simulink model "TTypeInverter_R2022a"  (R2022a)
settings: Solver=ode23t  StartTime=0.0  StopTime=0.2  RelTol=1e-3  EnableMultiTasking=on
values from neighbouring files (symbols this model uses):
  C_c = 30*10^-6    (= 3e-05)    [TTypeInverterVals.m]
  den = abs(G_pr_r_z.Denominator{1,1})    [TTypeInverterVals.m]
  den15 = abs(G_pr_r_15_z.Denominator{1,1})    [TTypeInverterVals.m]
  den21 = abs(G_pr_r_21_z.Denominator{1,1})    [TTypeInverterVals.m]
  den5 = abs(G_pr_r_5_z.Denominator{1,1})    [TTypeInverterVals.m]
  den7 = abs(G_pr_r_7_z.Denominator{1,1})    [TTypeInverterVals.m]
  f_o = 50    [TTypeInverterVals.m]
  G_diff_z = c2d(G_diff_s,Ts,opt)    [ControllerDesign.m]    (also in TTypeInverterVals.m = c2d(G_diff_s,Ts,'foh'))
  Kc = 2.5    [ControllerDesign.m]    (also in TTypeInverterVals.m)
  Klim = 5    [TTypeInverterVals.m]
  Kp = 1/mag/(10^(1.14/20))    [ControllerDesign.m]    (also in TTypeInverterVals.m = 0.9444)
  Kr = omega_c_o/2    (= 3141.59265359)    [ControllerDesign.m]    (also in TTypeInverterVals.m)
  N = 26    [Inductance.m]    (also in TTypeInverterVals.m = [0])
  num = abs(G_pr_r_z.Numerator{1,1})    [TTypeInverterVals.m]
  num15 = abs(G_pr_r_15_z.Numerator{1,1})    [TTypeInverterVals.m]
  num21 = abs(G_pr_r_21_z.Numerator{1,1})    [TTypeInverterVals.m]
  num5 = abs(G_pr_r_5_z.Numerator{1,1})    [TTypeInverterVals.m]
  num7 = abs(G_pr_r_7_z.Numerator{1,1})    [TTypeInverterVals.m]
  omega_o = fo*2*pi    (= 314.159265359)    [ControllerDesign.m]    (also in TTypeInverterVals.m)
  omega_w = 0.1*2*pi    (= 0.628318530718)    [ControllerDesign.m]    (also in TTypeInverterVals.m)
  pr_sat_val = ceil(3*io_nom)    [TTypeInverterVals.m]
  Q = eye(3)    [TTypeInverterVals.m]
  R = [R_iL 0 ... (first row only)    [TTypeInverterVals.m]
  R_l_20p = Vout^2/P_lin_20p    (= 10.58)    [TTypeInverterVals.m]
  R_l_3p = Vout/(P_max_3p/(Vout*3))    (= 2.116)    [TTypeInverterVals.m]
  R_l_80p = Vout^2/P_lin_80p    (= 2.645)    [TTypeInverterVals.m]
  R_l_nl = Vout^2/P_lin    (= 3.11176470588)    [TTypeInverterVals.m]
  R_l_nl_3p = Vout_3p^2/P_lin_3p    [TTypeInverterVals.m]
  R_Lc = 5.6e-3    (= 0.0056)    [TTypeInverterVals.m]
  R_nl_load = Uc^2/(0.66*S_tot)    (= 14.9121893939)    [TTypeInverterVals.m]
  R_nl_load_3p = Uc_3p^2/(0.66*S_tot_3p)    (= 4.97072979798)    [TTypeInverterVals.m]
  R_nl_s = 0.04*Vout^2/S_tot    (= 0.2645)    [TTypeInverterVals.m]
  R_nl_s_3p = 0.04*Vout_3p^2/S_tot_3p    [TTypeInverterVals.m]
  T_sw = 1/f_sw    (= 4.16666666667e-05)    [TTypeInverterVals.m]
  Tcomp = Ts/4    (= 2.60400009204e-06)    [TTypeInverterVals.m]
  Ts = 1/fs    (= 1.04166666667e-05)    [ControllerDesign.m]    (also in KalmanFilter.m = 2.08333333333e-05; TTypeInverterVals.m = 1.04160003681e-05)
  VDC = 800    [TTypeInverterVals.m]
  Vout_amp = Vout*sqrt(2)    [TTypeInverterVals.m]
undefined symbols (not defined in the file or in its folder): a0, a1, b0, b1, Discrete, G_ll_z, Ki, Kpc, KT, kv, Time, UKF_data
libraries: ee_lib x94, nesl_utility x48, fl_lib x39, dspstat3 x15, spsTriangleGeneratorLib x6, ctrlSharedLib x3, spsRMSLib x3, spsTHDLib x3
(part 1 of 5)
settings Model: Creator=sebastian  LastModifiedBy=sebastian
settings DataIOCC: ReturnWorkspaceOutputs=off
settings SimscapeCC: SimscapeNormalizeSystem=off

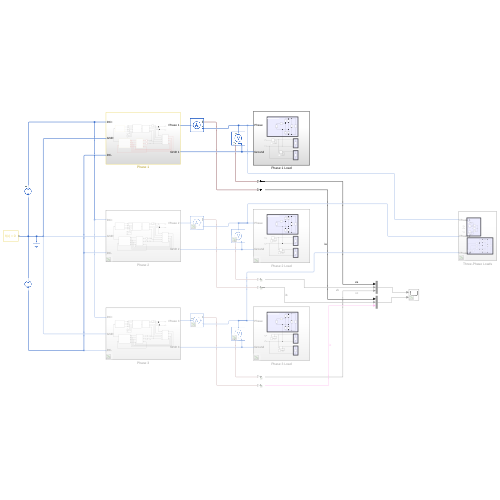
[thumbnail: Simulink's stored preview of the top-level diagram]
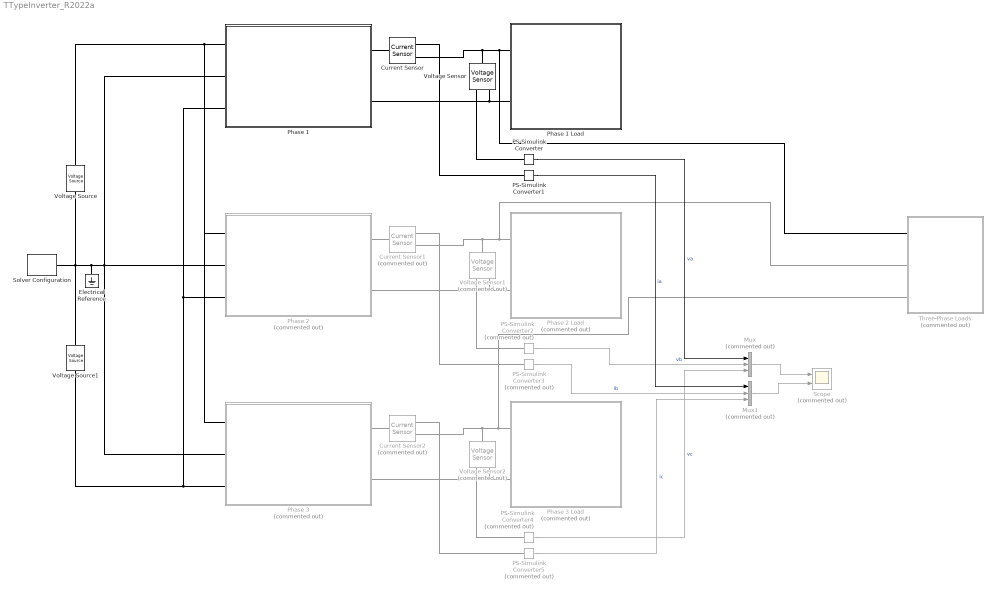
== system TTypeInverter_R2022a ==
  Current Sensor : fl_lib/Electrical/Electrical Sensors/Current Sensor
      settings: SourceProductBaseCode=PW,SS,VE
  Current Sensor1 : fl_lib/Electrical/Electrical Sensors/Current Sensor  Commented=on
      settings: SourceProductBaseCode=PW,SS,VE
  Current Sensor2 : fl_lib/Electrical/Electrical Sensors/Current Sensor  Commented=on
      settings: SourceProductBaseCode=PW,SS,VE
  Electrical Reference : fl_lib/Electrical/Electrical Elements/Electrical Reference
      settings: SourceProductBaseCode=PW,SS,VE
  Mux : Mux  Commented=on  Inputs=3
  Mux1 : Mux  Commented=on  Inputs=3
  PS-Simulink Converter : nesl_utility/PS-Simulink Converter  PhysicalDomain=network_engine_domain  SubClassName=ps_output  LeftPortType=input  RightPortType=output  PseudoPeriodic=off  Frequencies=[]  VectorFormat=inherit  Unit=inherit  AffineConversion=off
      settings: SourceProductBaseCode=SS,PW,VE
  PS-Simulink Converter1 : nesl_utility/PS-Simulink Converter  PhysicalDomain=network_engine_domain  SubClassName=ps_output  LeftPortType=input  RightPortType=output  PseudoPeriodic=off  Frequencies=[]  VectorFormat=inherit  Unit=inherit  AffineConversion=off
      settings: SourceProductBaseCode=SS,PW,VE
  PS-Simulink Converter{2..5} (4 alike) : nesl_utility/PS-Simulink Converter  Commented=on  PhysicalDomain=network_engine_domain  SubClassName=ps_output  LeftPortType=input  RightPortType=output  PseudoPeriodic=off  Frequencies=[]  VectorFormat=inherit  Unit=inherit  AffineConversion=off
      settings: SourceProductBaseCode=SS,PW,VE
  Phase 1 : Subsystem
  Phase 1 Load : Subsystem
  Phase 2 : Subsystem  Commented=on
  Phase 2 Load : Subsystem  Commented=on
  Phase 3 : Subsystem  Commented=on
  Phase 3 Load : Subsystem  Commented=on
  Scope : Scope  Commented=on  NumInputPorts=2
  Solver Configuration : nesl_utility/Solver Configuration  PhysicalDomain=network_engine_domain  SubClassName=solver  LeftPortType=input  RightPortType=generic  Tones=[]  Harmonics=[]  SimulateNoise=off  Profile=off  UseLocalSampling=off  EnableSwitchedLinearOptims=on  FrequencyDomain=off  UseCCode=off  RelTol=0.001  AbsTol=0.001  MinStep=1e-09  ToWorkspace=off  RevertToSquareIcSolve=off  NumHomotopyIterations=100  PhasorMode=off  PhasorModeNumHarmonics=1  IndexReductionMethod=DerivativeReplacement  DoDC=off  ResidualTolerance=1e-09  UseLocalSolver=off  LocalSolverChoice=NE_BACKWARD_EULER_ADVANCER  LocalSolverSampleTime=Ts/10000  DoFixedCost=off  MaxNonlinIter=3  MaxModeIter=2  ComputeImpulses=off  ImpulseIterations=2  LinearAlgebra=auto  LinearAlgebraNumThread=0  EquationFormulation=NE_TIME_EF  DelaysMemoryBudget=1024  AutomaticFiltering=on  FilteringTimeConstant=0.001  PartitionStorageMethod=AS_NEEDED  PartitionMemoryBudget=1024  PartitionMethod=ROBUST
      settings: SourceProductBaseCode=SS,PW,VE
  Three-Phase Loads : Subsystem  Commented=on
  Voltage Sensor : fl_lib/Electrical/Electrical Sensors/Voltage Sensor
      settings: SourceProductBaseCode=PW,SS,VE
  Voltage Sensor1 : fl_lib/Electrical/Electrical Sensors/Voltage Sensor  Commented=on
      settings: SourceProductBaseCode=PW,SS,VE
  Voltage Sensor2 : fl_lib/Electrical/Electrical Sensors/Voltage Sensor  Commented=on
      settings: SourceProductBaseCode=PW,SS,VE
  Voltage Source : ee_lib/Sources/Voltage Source  dc_voltage=VDC/2 V  ac_voltage=0 V  ac_shift=0 rad  ac_frequency=60 Hz  noise_mode=1  PSD=0.0001 V^2/Hz  repeatability=3  auto_seed=3437178441  user_seed=0  sample_time=Ts s  i_specify=off  i_priority=None  i=0 A  i_nominal_specify=off  i_nominal_unit=A  i_nominal_value=1  v_specify=off  v_priority=None  v=0 V  v_nominal_specify=off  v_nominal_unit=V  v_nominal_value=1
  Voltage Source1 : ee_lib/Sources/Voltage Source  dc_voltage=VDC/2 V  ac_voltage=0 V  ac_shift=0 rad  ac_frequency=60 Hz  noise_mode=1  PSD=0.0001 V^2/Hz  repeatability=3  auto_seed=609397185  user_seed=0  sample_time=Ts s  i_specify=off  i_priority=None  i=0 A  i_nominal_specify=off  i_nominal_unit=A  i_nominal_value=1  v_specify=off  v_priority=None  v=0 V  v_nominal_specify=off  v_nominal_unit=V  v_nominal_value=1
  wires:
  Mux/1 -> Scope/1
  Mux1/1 -> Scope/2
  PS-Simulink Converter/1 -> Mux/1  "va"
  PS-Simulink Converter2/1 -> Mux/2  "vb"
  PS-Simulink Converter4/1 -> Mux/3  "vc"
  PS-Simulink Converter1/1 -> Mux1/1  "ia"
  PS-Simulink Converter3/1 -> Mux1/2  "ib"
  PS-Simulink Converter5/1 -> Mux1/3  "ic"
  connections:
  Phase 1 Load/LConn2 -- Voltage Sensor/RConn2 -- Phase 1/RConn2
  Solver Configuration/RConn1 -- Phase 2/LConn2 -- Phase 3/LConn2 -- Phase 1/LConn2 -- Electrical Reference/LConn1 -- Voltage Source/RConn1 -- Voltage Source1/LConn1
  Voltage Source/LConn1 -- Phase 3/LConn1 -- Phase 2/LConn1 -- Phase 1/LConn1
  Phase 1/LConn3 -- Voltage Source1/RConn1 -- Phase 3/LConn3 -- Phase 2/LConn3
  Current Sensor/LConn1 -- Phase 1/RConn1
  Current Sensor/RConn2 -- Voltage Sensor/LConn1 -- Three-Phase Loads/LConn1 -- Phase 1 Load/LConn1
  PS-Simulink Converter/LConn1 -- Voltage Sensor/RConn1
  Current Sensor/RConn1 -- PS-Simulink Converter1/LConn1
  Current Sensor1/RConn2 -- Voltage Sensor1/LConn1 -- Three-Phase Loads/LConn2 -- Phase 2 Load/LConn1
  Phase 2 Load/LConn2 -- Voltage Sensor1/RConn2 -- Phase 2/RConn2
  PS-Simulink Converter2/LConn1 -- Voltage Sensor1/RConn1
  Current Sensor1/LConn1 -- Phase 2/RConn1
  Current Sensor1/RConn1 -- PS-Simulink Converter3/LConn1
  Current Sensor2/RConn2 -- Voltage Sensor2/LConn1 -- Three-Phase Loads/LConn3 -- Phase 3 Load/LConn1
  Phase 3 Load/LConn2 -- Voltage Sensor2/RConn2 -- Phase 3/RConn2
  PS-Simulink Converter4/LConn1 -- Voltage Sensor2/RConn1
  Current Sensor2/LConn1 -- Phase 3/RConn1
  Current Sensor2/RConn1 -- PS-Simulink Converter5/LConn1

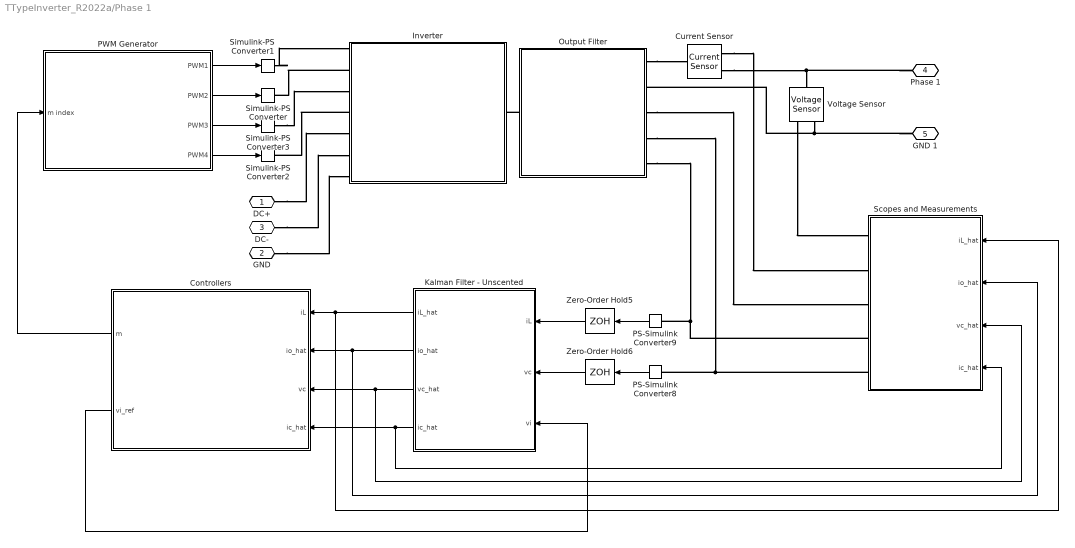
== system TTypeInverter_R2022a/Phase 1 ==
  Controllers : Subsystem
  Current Sensor : fl_lib/Electrical/Electrical Sensors/Current Sensor
      settings: SourceProductBaseCode=PW,SS,VE
  Inverter : Subsystem
  Kalman Filter - Unscented : Subsystem
  Output Filter : Subsystem
  PS-Simulink Converter8 : nesl_utility/PS-Simulink Converter  PhysicalDomain=network_engine_domain  SubClassName=ps_output  LeftPortType=input  RightPortType=output  PseudoPeriodic=off  Frequencies=[]  VectorFormat=inherit  Unit=inherit  AffineConversion=off
      settings: SourceProductBaseCode=SS,PW,VE
  PS-Simulink Converter9 : nesl_utility/PS-Simulink Converter  PhysicalDomain=network_engine_domain  SubClassName=ps_output  LeftPortType=input  RightPortType=output  PseudoPeriodic=off  Frequencies=[]  VectorFormat=inherit  Unit=inherit  AffineConversion=off
      settings: SourceProductBaseCode=SS,PW,VE
  PWM Generator : Subsystem
  Scopes and Measurements : Subsystem
      settings: PortSchema="{\"entries\":[{\"content\":{\"sides\":[{\"content\":{\"connectorIds\":[\"LConn1\",\"LConn2\",\"LConn3\",\"LConn4\",\"LConn5\"]},\"type\":\"ConnectorPlacement.EquallySpacedRectSide\",\"uuid\":\"9cb3f6d1-a698-4256-82c6-cde7349a629b\"},{\"content\":{\"connectorIds\":[\"In1\",\"In2\",\"In3\",\"In4\"],\"side\":\"RIGHT\"},\"type\":\"ConnectorPlacement.EquallySpacedRectSide\",\"uuid\":\"1e882b0f-d5eb-4cef-9b33-a811b5aef736\"},{\"content\":{\"connectorIds\":[],\"side\":\"TOP\"},\"type\":\"ConnectorPlacement.EquallySpacedRectSide\",\"uuid\":\"e9e8da66-95e1-4884-9361-97f2ef91d9a4\"}]},\"type\":\"ConnectorPlacement.EquallySpacedConnector\",\"uuid\":\"50359238-0e1d-4354-ac1b-c407791d07c2\"}],\"packageUris\":[\"http://schema.mathworks.com/mf0/Connector/R2020b\"],\"version\":\"1.0\"}"
  Simulink-PS Converter{,1..3} (4 alike) : nesl_utility/Simulink-PS Converter  PhysicalDomain=network_engine_domain  SubClassName=ps_input  LeftPortType=input  RightPortType=output  PseudoPeriodic=off  Frequencies=[]  NoiseDistribution=none  NoiseParameters=[]  Unit=1  AffineConversion=off  FilteringAndDerivatives=provide  SimscapeFilterOrder=1  InputFilterTimeConstant=0.001  UdotUserProvided=0
      settings: SourceProductBaseCode=SS,PW,VE
  Voltage Sensor : fl_lib/Electrical/Electrical Sensors/Voltage Sensor
      settings: SourceProductBaseCode=PW,SS,VE
  Zero-Order Hold5 : ZeroOrderHold  SampleTime=Ts
  Zero-Order Hold6 : ZeroOrderHold  SampleTime=Ts
  DC+ : PMIOPort  Side=Left
  GND : PMIOPort  Port=2  Side=Left
  DC- : PMIOPort  Port=3  Side=Left
  Phase 1 : PMIOPort  Port=4  Side=Right
  GND 1 : PMIOPort  Port=5  Side=Right
  wires:
  PS-Simulink Converter8/1 -> Zero-Order Hold6/1
  Kalman Filter - Unscented/1(iL_hat) -> Controllers/1(iL), Scopes and Measurements/1(iL_hat)
  PWM Generator/4(PWM4) -> Simulink-PS Converter2/1
  Controllers/2(vi_ref) -> Kalman Filter - Unscented/3(vi)
  Kalman Filter - Unscented/3(vc_hat) -> Scopes and Measurements/3(vc_hat), Controllers/3(vc)
  Zero-Order Hold5/1 -> Kalman Filter - Unscented/1(iL)
  PS-Simulink Converter9/1 -> Zero-Order Hold5/1
  Controllers/1(m) -> PWM Generator/1(m index)
  PWM Generator/2(PWM2) -> Simulink-PS Converter/1
  Zero-Order Hold6/1 -> Kalman Filter - Unscented/2(vc)
  PWM Generator/1(PWM1) -> Simulink-PS Converter1/1
  PWM Generator/3(PWM3) -> Simulink-PS Converter3/1
  Kalman Filter - Unscented/2(io_hat) -> Scopes and Measurements/2(io_hat), Controllers/2(io_hat)
  Kalman Filter - Unscented/4(ic_hat) -> Scopes and Measurements/4(ic_hat), Controllers/4(ic_hat)
  connections:
  Simulink-PS Converter3/RConn1 -- Inverter/LConn3
  Simulink-PS Converter1/RConn1 -- Inverter/LConn1
  Output Filter/RConn3 -- Scopes and Measurements/LConn3
  Voltage Sensor/RConn2 -- GND 1/RConn1 -- Output Filter/RConn2
  Voltage Sensor/RConn1 -- Scopes and Measurements/LConn1
  Current Sensor/RConn2 -- Phase 1/RConn1 -- Voltage Sensor/LConn1
  Inverter/LConn4 -- Simulink-PS Converter2/RConn1
  Output Filter/RConn5 -- Scopes and Measurements/LConn4 -- PS-Simulink Converter9/LConn1
  Output Filter/LConn1 -- Inverter/RConn1
  Current Sensor/RConn1 -- Scopes and Measurements/LConn2
  Inverter/LConn2 -- Simulink-PS Converter/RConn1
  Output Filter/RConn4 -- Scopes and Measurements/LConn5 -- PS-Simulink Converter8/LConn1
  Output Filter/RConn1 -- Current Sensor/LConn1
  DC+/RConn1 -- Inverter/LConn5
  DC-/RConn1 -- Inverter/LConn6
  GND/RConn1 -- Inverter/LConn7

== system TTypeInverter_R2022a/Phase 1 Load ==
  note: Capacitor may be pre-charged to 290V!
  note: Reference test load
  note: Reference nonlinear load
  note: 20% Load
  note: 80% Load
  Capacitor4 : ee_lib/Passive/Capacitor  cap_option=0  c=C_nl F  Cvec=[1e-05, 1e-06] F  Vvec=[0, 10] V  CV_table_symmetry=1  f_vec=[1, 10] kHz  DFext_vec=[.8, 1.2]  enable_C_tol=0  C_tol=5  tol_distribution=1  nSigma=4  r=R_C_nl Ohm  g=0 1/Ohm  averaging_period=0 s  enable_operating_limits=0  operating_limit_action=2  max_working_voltage_range=[-25, 25] V  power_rating=1 W  enable_faults=0  fault_action=1  Cscale_faulted=100  R_faulted=1e-3 Ohm  G_faulted=0 1/Ohm  tau_fault=1e-3 s  enable_temporal_fault=0  t_fault=1 s  enable_behavioral_fault=0  max_permissible_voltage_range=[-100, 100] V  t_fail_on_voltage=1 s  i_specify=off  i_priority=None  i=0 A  i_nominal_specify=off  i_nominal_unit=A  i_nominal_value=1  v_specify=off  v_priority=High  v=325 V  v_nominal_specify=off  v_nominal_unit=V  v_nominal_value=325  vc_specify=off  vc_priority=High  vc=290 V  vc_nominal_specify=off  vc_nominal_unit=V  vc_nominal_value=325
  Diode{1..4} (4 alike) : ee_lib/Semiconductors & Converters/Diode  ModelType=ee.enum.diode.modelType.pwl  TableType=ee.enum.diode.tableType.IfMat  IfMat=[.07, .12, .19, 1.75, 4.24, 7.32, 11.2; .16, .3, .72, 2.14, 5.02, 8.35, 13.12] A  VfMat=[.9, 1.15, 1.25, 1.5, 1.75, 2.17, 2.6, 2.85; .58, .68, .75, 1.1, 1.38, 1.77, 2.27, 2.7] V  TjVec=[25, 125] degC  VfVec=[.5, .7, .9, 1.3, 1.7, 2.1, 2.5] V  IfVec=[.1, .2, .5, 1, 2, 4, 7, 10] A  Vf=V_f V  Ron=R_d Ohm  Goff=1e-8 S  prmExp=ee.enum.diode.expParam.useTwo  I12=[.0137, .545] A  V12=[.6, .7] V  RS=0 Ohm  Tmeas=25 degC  IS=1e-12 A  ec=1  I1=0.0137 A  V1=0.6 V  N_series=1  N_parallel=1  Rz=0.3 Ohm  BV=inf V  C_param=ee.enum.diode.capParam.fixed  CJ=5 pF  CJ0=5 pF  Vvec=[.1, 10, 100] V  Cvec=[3.5, 1, .4] pF  VJ=1 V  Mgrad=0.5  FC=0.5  Q_param=ee.enum.diode.recoveryParam.off  iRM=-7.15 A  iF=4 A  didt=-750 A/us  trr_factor=3  trr=115 ns  Qrr=150 nA*s  Vr=-600 V  Ls=150 nH  Erec=0.03 J  TT=50 ns  tau=100 ns  T_param=ee.enum.diode.temperatureParam.off  Tdevice=25 degC  I1_T2=0.245 A  V1_T2=0.5 V  IS_T2=1.25e-7 A  Tmeas2=125 degC  XTI_param=ee.enum.diode.xtiParam.pn  XTI=3  EG_param=ee.enum.diode.egapParam.material_si  EG=1.11 eV  dBVdT=0 V/K  enable_faults=simscape.enum.onoff.off  fault_action=simscape.enum.assert.action.none  fault_types=ee.enum.diode.faults.open  tau_fault=1e-3 s  IfMat_faulted=[.07, .12, .19, 1.75, 4.24, 7.32, 11.2; .16, .3, .72, 2.14, 4.02, 6.35, 9.12] A  VfMat_faulted=[.9, 1.15, 1.25, 1.5, 1.75, 2.17, 2.6, 2.85; .58, .68, .75, 1.1, 1.38, 1.77, 2.27, 2.7] V  VfVec_faulted=[.5, .7, .9, 1.3, 1.7, 2.1, 2.5] V  IfVec_faulted=[.1, .2, .5, 1, 2, 4, 7, 10] A  Ropen_faulted=1000 Ohm  Gshort_faulted=1000 1/Ohm  Vf_faulted=0.6 V  Ron_faulted=0.3 Ohm  Goff_faulted=1e-8 S  I12_faulted=[.0137, .545] A  V12_faulted=[.6, .7] V  IS_faulted=1e-12 A  ec_faulted=1  I1_faulted=0.0137 A  V1_faulted=0.6 V  RS_faulted=0 Ohm  Rz_faulted=0.3 Ohm  BV_faulted=inf V  Cscale_faulted=100  enable_temporal_fault=simscape.enum.onoff.off  t_fault=inf s  enable_behavioral_fault=simscape.enum.onoff.off  max_permissible_voltage=inf V  n_fail_on_voltage=1  max_permissible_current=inf A  t_fail_on_current=1 s  max_permissible_dVdt=inf V/s  enable_fault_input=simscape.enum.onoff.off  i_specify=off  i_priority=None  i=0 A  i_nominal_specify=off  i_nominal_unit=A  i_nominal_value=1  v_specify=off  v_priority=None  v=0 V  v_nominal_specify=off  v_nominal_unit=V  v_nominal_value=1  i_diode_specify=off  i_diode_priority=None  i_diode=0 A  i_diode_nominal_specify=off  i_diode_nominal_unit=A  i_diode_nominal_value=1  v_diode_specify=off  v_diode_priority=None  v_diode=0 V  v_diode_nominal_specify=off  v_diode_nominal_unit=V  v_diode_nominal_value=1  i_capacitor_specify=off  i_capacitor_priority=None  i_capacitor=0 A  i_capacitor_nominal_specify=off  i_capacitor_nominal_unit=A  i_capacitor_nominal_value=1  v_capacitor_specify=off  v_capacitor_priority=None  v_capacitor=0 V  v_capacitor_nominal_specify=off  v_capacitor_nominal_unit=V  v_capacitor_nominal_value=1  power_dissipated_specify=off  power_dissipated_priority=None  power_dissipated=0 W  power_dissipated_nominal_specify=off  power_dissipated_nominal_unit=W  power_dissipated_nominal_value=1  max_permissible_temperature=inf K  t_fail_on_temperature=1 s  thermal_network_parameterization=ee.enum.thermalNetworkTopology.junctionCase  Rth=[0, 10] K/W  Rth_Cauer=[1, 3, 10] K/W  Rth_Foster=[4, 6] K/W  thermal_mass_parameterization=ee.enum.thermalNetwork.timeconstant  thermal_mass=[0, 1] J/K  thermal_mass_Cauer=[.1, .3, 1] J/K  thermal_mass_Foster=[1.5, 3] J/K  thermal_time_constant=[0, 10] s  thermal_time_constant_Cauer=[1, 3, 10] s  thermal_time_constant_Foster=[6, 18] s  thermal_mass_initial_temperatures=[25, 25] degC  thermal_mass_initial_temperatures_Cauer=[25, 25, 25] degC  steadyState_Foster=simscape.enum.onoff.on  Tvec_initial_Foster=[25, 25, 25, 25] degC
  Line Resistor : ee_lib/Passive/Resistor  R=R_nl_s Ohm  enable_R_tol=0  R_tol=5  tol_distribution=1  nSigma=4  enable_operating_limits=0  operating_limit_action=2  max_working_voltage=100 V  power_rating=1 W  enable_faults=0  fault_action=1  R_faulted=inf Ohm  enable_temporal_fault=0  t_fault=1 s  enable_behavioral_fault=0  max_permissible_current=1 A  t_fail_on_current=1 s  noise_mode=0  sample_time=1e-3 s  repeatability=1  auto_seed=3922919431  user_seed=0  Tdevice=25 degC  power_derating_T1=70 degC  power_derating_T2=155 degC  operating_temperature_range_vec=[-50, 150] degC  alpha=3.93e-3 1/K  Tmeas=25 degC  thermal_mass=100 J/K  temperature_specify=off  temperature_priority=High  temperature=298.15 K  temperature_nominal_specify=off  temperature_nominal_unit=K  temperature_nominal_value=1
  Linear Load : ee_lib/Passive/Resistor  R=R_l_nl Ohm  enable_R_tol=0  R_tol=5  tol_distribution=1  nSigma=4  enable_operating_limits=0  operating_limit_action=2  max_working_voltage=100 V  power_rating=1 W  enable_faults=0  fault_action=1  R_faulted=inf Ohm  enable_temporal_fault=0  t_fault=1 s  enable_behavioral_fault=0  max_permissible_current=1 A  t_fail_on_current=1 s  noise_mode=0  sample_time=1e-3 s  repeatability=1  auto_seed=3499211588  user_seed=0  Tdevice=25 degC  power_derating_T1=70 degC  power_derating_T2=155 degC  operating_temperature_range_vec=[-50, 150] degC  alpha=3.93e-3 1/K  Tmeas=25 degC  thermal_mass=100 J/K  temperature_specify=off  temperature_priority=High  temperature=298.15 K  temperature_nominal_specify=off  temperature_nominal_unit=K  temperature_nominal_value=1
  Resistor : ee_lib/Passive/Resistor  R=R_l_20p/5 Ohm  enable_R_tol=0  R_tol=5  tol_distribution=1  nSigma=4  enable_operating_limits=0  operating_limit_action=2  max_working_voltage=100 V  power_rating=1 W  enable_faults=0  fault_action=1  R_faulted=inf Ohm  enable_temporal_fault=0  t_fault=1 s  enable_behavioral_fault=0  max_permissible_current=1 A  t_fail_on_current=1 s  noise_mode=0  sample_time=1e-3 s  repeatability=1  auto_seed=3499211588  user_seed=0  Tdevice=25 degC  power_derating_T1=70 degC  power_derating_T2=155 degC  operating_temperature_range_vec=[-50, 150] degC  alpha=3.93e-3 1/K  Tmeas=25 degC  thermal_mass=100 J/K  temperature_specify=off  temperature_priority=High  temperature=298.15 K  temperature_nominal_specify=off  temperature_nominal_unit=K  temperature_nominal_value=1
  Resistor1 : ee_lib/Passive/Resistor  R=R_nl_load Ohm  enable_R_tol=0  R_tol=5  tol_distribution=1  nSigma=4  enable_operating_limits=0  operating_limit_action=2  max_working_voltage=100 V  power_rating=1 W  enable_faults=0  fault_action=1  R_faulted=inf Ohm  enable_temporal_fault=0  t_fault=1 s  enable_behavioral_fault=0  max_permissible_current=1 A  t_fail_on_current=1 s  noise_mode=0  sample_time=1e-3 s  repeatability=1  auto_seed=3499211588  user_seed=0  Tdevice=25 degC  power_derating_T1=70 degC  power_derating_T2=155 degC  operating_temperature_range_vec=[-50, 150] degC  alpha=3.93e-3 1/K  Tmeas=25 degC  thermal_mass=100 J/K  temperature_specify=off  temperature_priority=High  temperature=298.15 K  temperature_nominal_specify=off  temperature_nominal_unit=K  temperature_nominal_value=1
  Resistor3 : ee_lib/Passive/Resistor  R=R_l_80p/5 Ohm  enable_R_tol=0  R_tol=5  tol_distribution=1  nSigma=4  enable_operating_limits=0  operating_limit_action=2  max_working_voltage=100 V  power_rating=1 W  enable_faults=0  fault_action=1  R_faulted=inf Ohm  enable_temporal_fault=0  t_fault=1 s  enable_behavioral_fault=0  max_permissible_current=1 A  t_fail_on_current=1 s  noise_mode=0  sample_time=1e-3 s  repeatability=1  auto_seed=3922919431  user_seed=0  Tdevice=25 degC  power_derating_T1=70 degC  power_derating_T2=155 degC  operating_temperature_range_vec=[-50, 150] degC  alpha=3.93e-3 1/K  Tmeas=25 degC  thermal_mass=100 J/K  temperature_specify=off  temperature_priority=High  temperature=298.15 K  temperature_nominal_specify=off  temperature_nominal_unit=K  temperature_nominal_value=1
  Simulink-PS Converter4 : nesl_utility/Simulink-PS Converter  PhysicalDomain=network_engine_domain  SubClassName=ps_input  LeftPortType=input  RightPortType=output  PseudoPeriodic=off  Frequencies=[]  NoiseDistribution=none  NoiseParameters=[]  Unit=1  AffineConversion=off  FilteringAndDerivatives=provide  SimscapeFilterOrder=1  InputFilterTimeConstant=0.001  UdotUserProvided=0
      settings: SourceProductBaseCode=SS,PW,VE
  Simulink-PS Converter5 : nesl_utility/Simulink-PS Converter  PhysicalDomain=network_engine_domain  SubClassName=ps_input  LeftPortType=input  RightPortType=output  PseudoPeriodic=off  Frequencies=[]  NoiseDistribution=none  NoiseParameters=[]  Unit=1  AffineConversion=off  FilteringAndDerivatives=provide  SimscapeFilterOrder=1  InputFilterTimeConstant=0.001  UdotUserProvided=0
      settings: SourceProductBaseCode=SS,PW,VE
  Step : Step  Time=0.025  SampleTime=0
  Step1 : Step  Time=0.045  Before=1  After=0  SampleTime=0
  Switch : fl_lib/Electrical/Electrical Elements/Switch  R_closed=1e-9 Ohm  G_open=1e-12 1/Ohm  Threshold=0.5  i_specify=off  i_priority=None  i=0 A  i_nominal_specify=off  i_nominal_unit=A  i_nominal_value=1  v_specify=off  v_priority=None  v=0 V  v_nominal_specify=off  v_nominal_unit=V  v_nominal_value=1
      settings: SourceProductBaseCode=PW,SS,VE
  Switch1 : fl_lib/Electrical/Electrical Elements/Switch  R_closed=1e-9 Ohm  G_open=1e-12 1/Ohm  Threshold=0.5  i_specify=off  i_priority=None  i=0 A  i_nominal_specify=off  i_nominal_unit=A  i_nominal_value=1  v_specify=off  v_priority=None  v=0 V  v_nominal_specify=off  v_nominal_unit=V  v_nominal_value=1
      settings: SourceProductBaseCode=PW,SS,VE
  Phase : PMIOPort  Side=Left
  Ground : PMIOPort  Port=2  Side=Left
  wires:
  Step/1 -> Simulink-PS Converter4/1
  Step1/1 -> Simulink-PS Converter5/1
  connections:
  Simulink-PS Converter4/RConn1 -- Switch/RConn1
  Switch1/RConn1 -- Simulink-PS Converter5/RConn1
  Resistor3/LConn1 -- Switch1/RConn2
  Resistor1/LConn1 -- Capacitor4/LConn1 -- Diode4/RConn1 -- Diode1/RConn1
  Diode3/RConn1 -- Ground/RConn1 -- Resistor3/RConn1 -- Resistor/RConn1 -- Linear Load/RConn1 -- Diode1/LConn1
  Diode2/LConn1 -- Resistor1/RConn1 -- Capacitor4/RConn1 -- Diode3/LConn1
  Line Resistor/RConn1 -- Diode2/RConn1 -- Diode4/LConn1
  Switch1/LConn1 -- Switch/RConn2 -- Resistor/LConn1
  Linear Load/LConn1 -- Line Resistor/LConn1
  Phase/RConn1 -- Switch/LConn1

== system TTypeInverter_R2022a/Phase 2 ==
  Controllers : Subsystem
  Current Sensor : fl_lib/Electrical/Electrical Sensors/Current Sensor
      settings: SourceProductBaseCode=PW,SS,VE
  Inverter : Subsystem
  Kalman Filter - Unscented : Subsystem
  Output Filter : Subsystem
  PS-Simulink Converter8 : nesl_utility/PS-Simulink Converter  PhysicalDomain=network_engine_domain  SubClassName=ps_output  LeftPortType=input  RightPortType=output  PseudoPeriodic=off  Frequencies=[]  VectorFormat=inherit  Unit=inherit  AffineConversion=off
      settings: SourceProductBaseCode=SS,PW,VE
  PS-Simulink Converter9 : nesl_utility/PS-Simulink Converter  PhysicalDomain=network_engine_domain  SubClassName=ps_output  LeftPortType=input  RightPortType=output  PseudoPeriodic=off  Frequencies=[]  VectorFormat=inherit  Unit=inherit  AffineConversion=off
      settings: SourceProductBaseCode=SS,PW,VE
  PWM Generator : Subsystem
  Scopes and Measurements : Subsystem
      settings: PortSchema="{\"entries\":[{\"content\":{\"sides\":[{\"content\":{\"connectorIds\":[\"LConn1\",\"LConn2\",\"LConn3\",\"LConn4\",\"LConn5\"]},\"type\":\"ConnectorPlacement.EquallySpacedRectSide\",\"uuid\":\"9cb3f6d1-a698-4256-82c6-cde7349a629b\"},{\"content\":{\"connectorIds\":[\"In1\",\"In2\",\"In3\",\"In4\"],\"side\":\"RIGHT\"},\"type\":\"ConnectorPlacement.EquallySpacedRectSide\",\"uuid\":\"1e882b0f-d5eb-4cef-9b33-a811b5aef736\"},{\"content\":{\"connectorIds\":[],\"side\":\"TOP\"},\"type\":\"ConnectorPlacement.EquallySpacedRectSide\",\"uuid\":\"e9e8da66-95e1-4884-9361-97f2ef91d9a4\"}]},\"type\":\"ConnectorPlacement.EquallySpacedConnector\",\"uuid\":\"50359238-0e1d-4354-ac1b-c407791d07c2\"}],\"packageUris\":[\"http://schema.mathworks.com/mf0/Connector/R2020b\"],\"version\":\"1.0\"}"
  Simulink-PS Converter{,1..3} (4 alike) : nesl_utility/Simulink-PS Converter  PhysicalDomain=network_engine_domain  SubClassName=ps_input  LeftPortType=input  RightPortType=output  PseudoPeriodic=off  Frequencies=[]  NoiseDistribution=none  NoiseParameters=[]  Unit=1  AffineConversion=off  FilteringAndDerivatives=provide  SimscapeFilterOrder=1  InputFilterTimeConstant=0.001  UdotUserProvided=0
      settings: SourceProductBaseCode=SS,PW,VE
  Voltage Sensor : fl_lib/Electrical/Electrical Sensors/Voltage Sensor
      settings: SourceProductBaseCode=PW,SS,VE
  Zero-Order Hold5 : ZeroOrderHold  SampleTime=Ts
  Zero-Order Hold6 : ZeroOrderHold  SampleTime=Ts
  DC+ : PMIOPort  Side=Left
  GND : PMIOPort  Port=2  Side=Left
  DC- : PMIOPort  Port=3  Side=Left
  Phase 2 : PMIOPort  Port=4  Side=Right
  GND 2 : PMIOPort  Port=5  Side=Right
  wires:
  PS-Simulink Converter8/1 -> Zero-Order Hold6/1
  Kalman Filter - Unscented/1(iL_hat) -> Controllers/1(iL), Scopes and Measurements/1(iL_hat)
  PWM Generator/4(PWM4) -> Simulink-PS Converter2/1
  Controllers/2(vi_ref) -> Kalman Filter - Unscented/3(vi)
  Kalman Filter - Unscented/3(vc_hat) -> Scopes and Measurements/3(vc_hat), Controllers/3(vc)
  Zero-Order Hold5/1 -> Kalman Filter - Unscented/1(iL)
  PS-Simulink Converter9/1 -> Zero-Order Hold5/1
  Controllers/1(m) -> PWM Generator/1(m index)
  PWM Generator/2(PWM2) -> Simulink-PS Converter/1
  Zero-Order Hold6/1 -> Kalman Filter - Unscented/2(vc)
  PWM Generator/1(PWM1) -> Simulink-PS Converter1/1
  PWM Generator/3(PWM3) -> Simulink-PS Converter3/1
  Kalman Filter - Unscented/2(io_hat) -> Scopes and Measurements/2(io_hat), Controllers/2(io_hat)
  Kalman Filter - Unscented/4(ic_hat) -> Scopes and Measurements/4(ic_hat), Controllers/4(ic_hat)
  connections:
  Simulink-PS Converter3/RConn1 -- Inverter/LConn3
  Simulink-PS Converter1/RConn1 -- Inverter/LConn1
  Output Filter/RConn3 -- Scopes and Measurements/LConn3
  Voltage Sensor/RConn2 -- Output Filter/RConn2 -- GND 2/RConn1
  Voltage Sensor/RConn1 -- Scopes and Measurements/LConn1
  Current Sensor/RConn2 -- Voltage Sensor/LConn1 -- Phase 2/RConn1
  Inverter/LConn4 -- Simulink-PS Converter2/RConn1
  Output Filter/RConn5 -- Scopes and Measurements/LConn4 -- PS-Simulink Converter9/LConn1
  Output Filter/LConn1 -- Inverter/RConn1
  Current Sensor/RConn1 -- Scopes and Measurements/LConn2
  Inverter/LConn2 -- Simulink-PS Converter/RConn1
  Output Filter/RConn4 -- Scopes and Measurements/LConn5 -- PS-Simulink Converter8/LConn1
  Output Filter/RConn1 -- Current Sensor/LConn1
  DC+/RConn1 -- Inverter/LConn5
  DC-/RConn1 -- Inverter/LConn6
  GND/RConn1 -- Inverter/LConn7

== system TTypeInverter_R2022a/Phase 2 Load ==
  note: Capacitor may be pre-charged to 290V!
  note: Reference test load
  note: Reference nonlinear load
  note: 20% Load
  note: 80% Load
  Capacitor4 : ee_lib/Passive/Capacitor  cap_option=0  c=C_nl F  Cvec=[1e-05, 1e-06] F  Vvec=[0, 10] V  CV_table_symmetry=1  f_vec=[1, 10] kHz  DFext_vec=[.8, 1.2]  enable_C_tol=0  C_tol=5  tol_distribution=1  nSigma=4  r=R_C_nl Ohm  g=0 1/Ohm  averaging_period=0 s  enable_operating_limits=0  operating_limit_action=2  max_working_voltage_range=[-25, 25] V  power_rating=1 W  enable_faults=0  fault_action=1  Cscale_faulted=100  R_faulted=1e-3 Ohm  G_faulted=0 1/Ohm  tau_fault=1e-3 s  enable_temporal_fault=0  t_fault=1 s  enable_behavioral_fault=0  max_permissible_voltage_range=[-100, 100] V  t_fail_on_voltage=1 s  i_specify=off  i_priority=None  i=0 A  i_nominal_specify=off  i_nominal_unit=A  i_nominal_value=1  v_specify=off  v_priority=High  v=325 V  v_nominal_specify=off  v_nominal_unit=V  v_nominal_value=325  vc_specify=off  vc_priority=High  vc=290 V  vc_nominal_specify=off  vc_nominal_unit=V  vc_nominal_value=325
  Diode{1..4} (4 alike) : ee_lib/Semiconductors & Converters/Diode  ModelType=ee.enum.diode.modelType.pwl  TableType=ee.enum.diode.tableType.IfMat  IfMat=[.07, .12, .19, 1.75, 4.24, 7.32, 11.2; .16, .3, .72, 2.14, 5.02, 8.35, 13.12] A  VfMat=[.9, 1.15, 1.25, 1.5, 1.75, 2.17, 2.6, 2.85; .58, .68, .75, 1.1, 1.38, 1.77, 2.27, 2.7] V  TjVec=[25, 125] degC  VfVec=[.5, .7, .9, 1.3, 1.7, 2.1, 2.5] V  IfVec=[.1, .2, .5, 1, 2, 4, 7, 10] A  Vf=V_f V  Ron=R_d Ohm  Goff=1e-8 S  prmExp=ee.enum.diode.expParam.useTwo  I12=[.0137, .545] A  V12=[.6, .7] V  RS=0 Ohm  Tmeas=25 degC  IS=1e-12 A  ec=1  I1=0.0137 A  V1=0.6 V  N_series=1  N_parallel=1  Rz=0.3 Ohm  BV=inf V  C_param=ee.enum.diode.capParam.fixed  CJ=5 pF  CJ0=5 pF  Vvec=[.1, 10, 100] V  Cvec=[3.5, 1, .4] pF  VJ=1 V  Mgrad=0.5  FC=0.5  Q_param=ee.enum.diode.recoveryParam.off  iRM=-7.15 A  iF=4 A  didt=-750 A/us  trr_factor=3  trr=115 ns  Qrr=150 nA*s  Vr=-600 V  Ls=150 nH  Erec=0.03 J  TT=50 ns  tau=100 ns  T_param=ee.enum.diode.temperatureParam.off  Tdevice=25 degC  I1_T2=0.245 A  V1_T2=0.5 V  IS_T2=1.25e-7 A  Tmeas2=125 degC  XTI_param=ee.enum.diode.xtiParam.pn  XTI=3  EG_param=ee.enum.diode.egapParam.material_si  EG=1.11 eV  dBVdT=0 V/K  enable_faults=simscape.enum.onoff.off  fault_action=simscape.enum.assert.action.none  fault_types=ee.enum.diode.faults.open  tau_fault=1e-3 s  IfMat_faulted=[.07, .12, .19, 1.75, 4.24, 7.32, 11.2; .16, .3, .72, 2.14, 4.02, 6.35, 9.12] A  VfMat_faulted=[.9, 1.15, 1.25, 1.5, 1.75, 2.17, 2.6, 2.85; .58, .68, .75, 1.1, 1.38, 1.77, 2.27, 2.7] V  VfVec_faulted=[.5, .7, .9, 1.3, 1.7, 2.1, 2.5] V  IfVec_faulted=[.1, .2, .5, 1, 2, 4, 7, 10] A  Ropen_faulted=1000 Ohm  Gshort_faulted=1000 1/Ohm  Vf_faulted=0.6 V  Ron_faulted=0.3 Ohm  Goff_faulted=1e-8 S  I12_faulted=[.0137, .545] A  V12_faulted=[.6, .7] V  IS_faulted=1e-12 A  ec_faulted=1  I1_faulted=0.0137 A  V1_faulted=0.6 V  RS_faulted=0 Ohm  Rz_faulted=0.3 Ohm  BV_faulted=inf V  Cscale_faulted=100  enable_temporal_fault=simscape.enum.onoff.off  t_fault=inf s  enable_behavioral_fault=simscape.enum.onoff.off  max_permissible_voltage=inf V  n_fail_on_voltage=1  max_permissible_current=inf A  t_fail_on_current=1 s  max_permissible_dVdt=inf V/s  enable_fault_input=simscape.enum.onoff.off  i_specify=off  i_priority=None  i=0 A  i_nominal_specify=off  i_nominal_unit=A  i_nominal_value=1  v_specify=off  v_priority=None  v=0 V  v_nominal_specify=off  v_nominal_unit=V  v_nominal_value=1  i_diode_specify=off  i_diode_priority=None  i_diode=0 A  i_diode_nominal_specify=off  i_diode_nominal_unit=A  i_diode_nominal_value=1  v_diode_specify=off  v_diode_priority=None  v_diode=0 V  v_diode_nominal_specify=off  v_diode_nominal_unit=V  v_diode_nominal_value=1  i_capacitor_specify=off  i_capacitor_priority=None  i_capacitor=0 A  i_capacitor_nominal_specify=off  i_capacitor_nominal_unit=A  i_capacitor_nominal_value=1  v_capacitor_specify=off  v_capacitor_priority=None  v_capacitor=0 V  v_capacitor_nominal_specify=off  v_capacitor_nominal_unit=V  v_capacitor_nominal_value=1  power_dissipated_specify=off  power_dissipated_priority=None  power_dissipated=0 W  power_dissipated_nominal_specify=off  power_dissipated_nominal_unit=W  power_dissipated_nominal_value=1  max_permissible_temperature=inf K  t_fail_on_temperature=1 s  thermal_network_parameterization=ee.enum.thermalNetworkTopology.junctionCase  Rth=[0, 10] K/W  Rth_Cauer=[1, 3, 10] K/W  Rth_Foster=[4, 6] K/W  thermal_mass_parameterization=ee.enum.thermalNetwork.timeconstant  thermal_mass=[0, 1] J/K  thermal_mass_Cauer=[.1, .3, 1] J/K  thermal_mass_Foster=[1.5, 3] J/K  thermal_time_constant=[0, 10] s  thermal_time_constant_Cauer=[1, 3, 10] s  thermal_time_constant_Foster=[6, 18] s  thermal_mass_initial_temperatures=[25, 25] degC  thermal_mass_initial_temperatures_Cauer=[25, 25, 25] degC  steadyState_Foster=simscape.enum.onoff.on  Tvec_initial_Foster=[25, 25, 25, 25] degC
  Line Resistor : ee_lib/Passive/Resistor  R=R_nl_s Ohm  enable_R_tol=0  R_tol=5  tol_distribution=1  nSigma=4  enable_operating_limits=0  operating_limit_action=2  max_working_voltage=100 V  power_rating=1 W  enable_faults=0  fault_action=1  R_faulted=inf Ohm  enable_temporal_fault=0  t_fault=1 s  enable_behavioral_fault=0  max_permissible_current=1 A  t_fail_on_current=1 s  noise_mode=0  sample_time=1e-3 s  repeatability=1  auto_seed=1811450916  user_seed=0  Tdevice=25 degC  power_derating_T1=70 degC  power_derating_T2=155 degC  operating_temperature_range_vec=[-50, 150] degC  alpha=3.93e-3 1/K  Tmeas=25 degC  thermal_mass=100 J/K  temperature_specify=off  temperature_priority=High  temperature=298.15 K  temperature_nominal_specify=off  temperature_nominal_unit=K  temperature_nominal_value=1
  Linear Load : ee_lib/Passive/Resistor  R=R_l_nl Ohm  enable_R_tol=0  R_tol=5  tol_distribution=1  nSigma=4  enable_operating_limits=0  operating_limit_action=2  max_working_voltage=100 V  power_rating=1 W  enable_faults=0  fault_action=1  R_faulted=inf Ohm  enable_temporal_fault=0  t_fault=1 s  enable_behavioral_fault=0  max_permissible_current=1 A  t_fail_on_current=1 s  noise_mode=0  sample_time=1e-3 s  repeatability=1  auto_seed=3933054132  user_seed=0  Tdevice=25 degC  power_derating_T1=70 degC  power_derating_T2=155 degC  operating_temperature_range_vec=[-50, 150] degC  alpha=3.93e-3 1/K  Tmeas=25 degC  thermal_mass=100 J/K  temperature_specify=off  temperature_priority=High  temperature=298.15 K  temperature_nominal_specify=off  temperature_nominal_unit=K  temperature_nominal_value=1
  Resistor : ee_lib/Passive/Resistor  R=R_l_20p Ohm  enable_R_tol=0  R_tol=5  tol_distribution=1  nSigma=4  enable_operating_limits=0  operating_limit_action=2  max_working_voltage=100 V  power_rating=1 W  enable_faults=0  fault_action=1  R_faulted=inf Ohm  enable_temporal_fault=0  t_fault=1 s  enable_behavioral_fault=0  max_permissible_current=1 A  t_fail_on_current=1 s  noise_mode=0  sample_time=1e-3 s  repeatability=1  auto_seed=3402504572  user_seed=0  Tdevice=25 degC  power_derating_T1=70 degC  power_derating_T2=155 degC  operating_temperature_range_vec=[-50, 150] degC  alpha=3.93e-3 1/K  Tmeas=25 degC  thermal_mass=100 J/K  temperature_specify=off  temperature_priority=High  temperature=298.15 K  temperature_nominal_specify=off  temperature_nominal_unit=K  temperature_nominal_value=1
  Resistor1 : ee_lib/Passive/Resistor  R=R_nl_load Ohm  enable_R_tol=0  R_tol=5  tol_distribution=1  nSigma=4  enable_operating_limits=0  operating_limit_action=2  max_working_voltage=100 V  power_rating=1 W  enable_faults=0  fault_action=1  R_faulted=inf Ohm  enable_temporal_fault=0  t_fault=1 s  enable_behavioral_fault=0  max_permissible_current=1 A  t_fail_on_current=1 s  noise_mode=0  sample_time=1e-3 s  repeatability=1  auto_seed=4120988592  user_seed=0  Tdevice=25 degC  power_derating_T1=70 degC  power_derating_T2=155 degC  operating_temperature_range_vec=[-50, 150] degC  alpha=3.93e-3 1/K  Tmeas=25 degC  thermal_mass=100 J/K  temperature_specify=off  temperature_priority=High  temperature=298.15 K  temperature_nominal_specify=off  temperature_nominal_unit=K  temperature_nominal_value=1
  Resistor3 : ee_lib/Passive/Resistor  R=R_l_80p Ohm  enable_R_tol=0  R_tol=5  tol_distribution=1  nSigma=4  enable_operating_limits=0  operating_limit_action=2  max_working_voltage=100 V  power_rating=1 W  enable_faults=0  fault_action=1  R_faulted=inf Ohm  enable_temporal_fault=0  t_fault=1 s  enable_behavioral_fault=0  max_permissible_current=1 A  t_fail_on_current=1 s  noise_mode=0  sample_time=1e-3 s  repeatability=1  auto_seed=2816384857  user_seed=0  Tdevice=25 degC  power_derating_T1=70 degC  power_derating_T2=155 degC  operating_temperature_range_vec=[-50, 150] degC  alpha=3.93e-3 1/K  Tmeas=25 degC  thermal_mass=100 J/K  temperature_specify=off  temperature_priority=High  temperature=298.15 K  temperature_nominal_specify=off  temperature_nominal_unit=K  temperature_nominal_value=1
  Simulink-PS Converter4 : nesl_utility/Simulink-PS Converter  PhysicalDomain=network_engine_domain  SubClassName=ps_input  LeftPortType=input  RightPortType=output  PseudoPeriodic=off  Frequencies=[]  NoiseDistribution=none  NoiseParameters=[]  Unit=1  AffineConversion=off  FilteringAndDerivatives=provide  SimscapeFilterOrder=1  InputFilterTimeConstant=0.001  UdotUserProvided=0
      settings: SourceProductBaseCode=SS,PW,VE
  Simulink-PS Converter5 : nesl_utility/Simulink-PS Converter  PhysicalDomain=network_engine_domain  SubClassName=ps_input  LeftPortType=input  RightPortType=output  PseudoPeriodic=off  Frequencies=[]  NoiseDistribution=none  NoiseParameters=[]  Unit=1  AffineConversion=off  FilteringAndDerivatives=provide  SimscapeFilterOrder=1  InputFilterTimeConstant=0.001  UdotUserProvided=0
      settings: SourceProductBaseCode=SS,PW,VE
  Step : Step  Time=0.025  SampleTime=0
  Step1 : Step  Time=0.025+1  Before=1  After=0  SampleTime=0
  Switch : fl_lib/Electrical/Electrical Elements/Switch  R_closed=1e-9 Ohm  G_open=1e-12 1/Ohm  Threshold=0.5  i_specify=off  i_priority=None  i=0 A  i_nominal_specify=off  i_nominal_unit=A  i_nominal_value=1  v_specify=off  v_priority=None  v=0 V  v_nominal_specify=off  v_nominal_unit=V  v_nominal_value=1
      settings: SourceProductBaseCode=PW,SS,VE
  Switch1 : fl_lib/Electrical/Electrical Elements/Switch  R_closed=1e-9 Ohm  G_open=1e-12 1/Ohm  Threshold=0.5  i_specify=off  i_priority=None  i=0 A  i_nominal_specify=off  i_nominal_unit=A  i_nominal_value=1  v_specify=off  v_priority=None  v=0 V  v_nominal_specify=off  v_nominal_unit=V  v_nominal_value=1
      settings: SourceProductBaseCode=PW,SS,VE
  Phase : PMIOPort  Side=Left
  Ground : PMIOPort  Port=2  Side=Left
  wires:
  Step/1 -> Simulink-PS Converter4/1
  Step1/1 -> Simulink-PS Converter5/1
  connections:
  Simulink-PS Converter4/RConn1 -- Switch/RConn1
  Switch1/RConn1 -- Simulink-PS Converter5/RConn1
  Resistor3/LConn1 -- Switch1/RConn2
  Resistor1/LConn1 -- Capacitor4/LConn1 -- Diode4/RConn1 -- Diode1/RConn1
  Diode3/RConn1 -- Ground/RConn1 -- Resistor3/RConn1 -- Resistor/RConn1 -- Linear Load/RConn1 -- Diode1/LConn1
  Diode2/LConn1 -- Resistor1/RConn1 -- Capacitor4/RConn1 -- Diode3/LConn1
  Line Resistor/RConn1 -- Diode2/RConn1 -- Diode4/LConn1
  Switch1/LConn1 -- Resistor/LConn1 -- Switch/RConn2
  Linear Load/LConn1 -- Line Resistor/LConn1

== system TTypeInverter_R2022a/Phase 3 ==
  Controllers : Subsystem
  Current Sensor : fl_lib/Electrical/Electrical Sensors/Current Sensor
      settings: SourceProductBaseCode=PW,SS,VE
  Inverter : Subsystem
  Kalman Filter - Unscented : Subsystem
  Output Filter : Subsystem
  PS-Simulink Converter8 : nesl_utility/PS-Simulink Converter  PhysicalDomain=network_engine_domain  SubClassName=ps_output  LeftPortType=input  RightPortType=output  PseudoPeriodic=off  Frequencies=[]  VectorFormat=inherit  Unit=inherit  AffineConversion=off
      settings: SourceProductBaseCode=SS,PW,VE
  PS-Simulink Converter9 : nesl_utility/PS-Simulink Converter  PhysicalDomain=network_engine_domain  SubClassName=ps_output  LeftPortType=input  RightPortType=output  PseudoPeriodic=off  Frequencies=[]  VectorFormat=inherit  Unit=inherit  AffineConversion=off
      settings: SourceProductBaseCode=SS,PW,VE
  PWM Generator : Subsystem
  Scopes and Measurements : Subsystem
      settings: PortSchema="{\"entries\":[{\"content\":{\"sides\":[{\"content\":{\"connectorIds\":[\"LConn1\",\"LConn2\",\"LConn3\",\"LConn4\",\"LConn5\"]},\"type\":\"ConnectorPlacement.EquallySpacedRectSide\",\"uuid\":\"9cb3f6d1-a698-4256-82c6-cde7349a629b\"},{\"content\":{\"connectorIds\":[\"In1\",\"In2\",\"In3\",\"In4\"],\"side\":\"RIGHT\"},\"type\":\"ConnectorPlacement.EquallySpacedRectSide\",\"uuid\":\"1e882b0f-d5eb-4cef-9b33-a811b5aef736\"},{\"content\":{\"connectorIds\":[],\"side\":\"TOP\"},\"type\":\"ConnectorPlacement.EquallySpacedRectSide\",\"uuid\":\"e9e8da66-95e1-4884-9361-97f2ef91d9a4\"}]},\"type\":\"ConnectorPlacement.EquallySpacedConnector\",\"uuid\":\"50359238-0e1d-4354-ac1b-c407791d07c2\"}],\"packageUris\":[\"http://schema.mathworks.com/mf0/Connector/R2020b\"],\"version\":\"1.0\"}"
  Simulink-PS Converter{,1..3} (4 alike) : nesl_utility/Simulink-PS Converter  PhysicalDomain=network_engine_domain  SubClassName=ps_input  LeftPortType=input  RightPortType=output  PseudoPeriodic=off  Frequencies=[]  NoiseDistribution=none  NoiseParameters=[]  Unit=1  AffineConversion=off  FilteringAndDerivatives=provide  SimscapeFilterOrder=1  InputFilterTimeConstant=0.001  UdotUserProvided=0
      settings: SourceProductBaseCode=SS,PW,VE
  Voltage Sensor : fl_lib/Electrical/Electrical Sensors/Voltage Sensor
      settings: SourceProductBaseCode=PW,SS,VE
  Zero-Order Hold5 : ZeroOrderHold  SampleTime=Ts
  Zero-Order Hold6 : ZeroOrderHold  SampleTime=Ts
  DC+ : PMIOPort  Side=Left
  GND : PMIOPort  Port=2  Side=Left
  DC- : PMIOPort  Port=3  Side=Left
  Phase 3 : PMIOPort  Port=4  Side=Right
  GND 3 : PMIOPort  Port=5  Side=Right
  wires:
  PS-Simulink Converter8/1 -> Zero-Order Hold6/1
  Kalman Filter - Unscented/1(iL_hat) -> Controllers/1(iL), Scopes and Measurements/1(iL_hat)
  PWM Generator/4(PWM4) -> Simulink-PS Converter2/1
  Controllers/2(vi_ref) -> Kalman Filter - Unscented/3(vi)
  Kalman Filter - Unscented/3(vc_hat) -> Scopes and Measurements/3(vc_hat), Controllers/3(vc)
  Zero-Order Hold5/1 -> Kalman Filter - Unscented/1(iL)
  PS-Simulink Converter9/1 -> Zero-Order Hold5/1
  Controllers/1(m) -> PWM Generator/1(m index)
  PWM Generator/2(PWM2) -> Simulink-PS Converter/1
  Zero-Order Hold6/1 -> Kalman Filter - Unscented/2(vc)
  PWM Generator/1(PWM1) -> Simulink-PS Converter1/1
  PWM Generator/3(PWM3) -> Simulink-PS Converter3/1
  Kalman Filter - Unscented/2(io_hat) -> Scopes and Measurements/2(io_hat), Controllers/2(io_hat)
  Kalman Filter - Unscented/4(ic_hat) -> Scopes and Measurements/4(ic_hat), Controllers/4(ic_hat)
  connections:
  Simulink-PS Converter3/RConn1 -- Inverter/LConn3
  Simulink-PS Converter1/RConn1 -- Inverter/LConn1
  Output Filter/RConn3 -- Scopes and Measurements/LConn3
  Voltage Sensor/RConn2 -- Output Filter/RConn2 -- GND 3/RConn1
  Voltage Sensor/RConn1 -- Scopes and Measurements/LConn1
  Current Sensor/RConn2 -- Voltage Sensor/LConn1 -- Phase 3/RConn1
  Inverter/LConn4 -- Simulink-PS Converter2/RConn1
  Output Filter/RConn5 -- Scopes and Measurements/LConn4 -- PS-Simulink Converter9/LConn1
  Output Filter/LConn1 -- Inverter/RConn1
  Current Sensor/RConn1 -- Scopes and Measurements/LConn2
  Inverter/LConn2 -- Simulink-PS Converter/RConn1
  Output Filter/RConn4 -- Scopes and Measurements/LConn5 -- PS-Simulink Converter8/LConn1
  Output Filter/RConn1 -- Current Sensor/LConn1
  DC+/RConn1 -- Inverter/LConn5
  DC-/RConn1 -- Inverter/LConn6
  GND/RConn1 -- Inverter/LConn7
